simulink model "baitap"  (R2018a)
settings: Solver=ode5  StartTime=0.0  StopTime=3  FixedStep=0.01  RelTol=1e-3
libraries: fuzblock x1
settings Model: Creator=DELL  LastModifiedBy=DELL

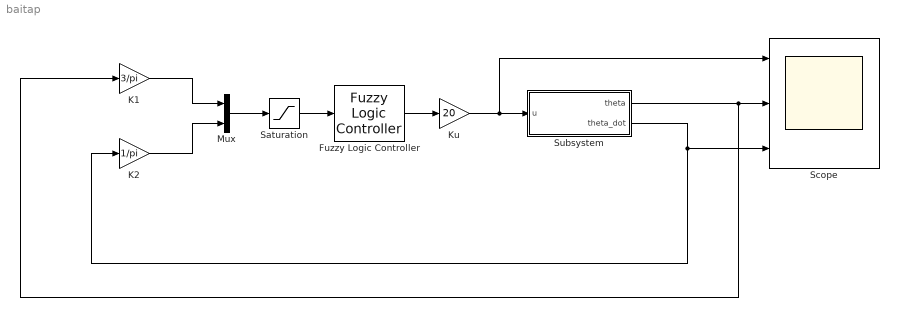
== system baitap ==
  Fuzzy Logic Controller : fuzblock/Fuzzy Logic  Controller  FIS='exex.fis'  OutputSampleNumber=101  DataType=double  FuzzifiedInputs=off  RuleFiringStrengths=off  RuleOutputs=off  AggregatedOutputs=off  SimulateUsing=Interpreted execution  OutOfRangeInputValueMessage=warning  NoRuleFiredMessage=warning  EmptyOutputFuzzySetMessage=warning
  "K1 " : Gain  Gain=3/pi
  "K2 " : Gain  Gain=1/pi
  "Ku " : Gain  Gain=20
  Mux : Mux  Inputs=2
  Saturation : Saturate  UpperLimit=1  LowerLimit=-1
  Scope : Scope  NumInputPorts=3
  Subsystem : Subsystem  mask{M1=1, m=0.1, g=9.81, l=0.5, theta_0=5, theta_dot_0=0}
      mask prompts: theta_0 "theta"; theta_dot_0 "theta_dot"
  wires:
  Saturation/1 -> Fuzzy Logic Controller/1
  Subsystem/1(theta) -> "K1 "/1, Scope/2
  Subsystem/2(theta_dot) -> Scope/3, "K2 "/1
  Fuzzy Logic Controller/1 -> "Ku "/1
  "Ku "/1 -> Subsystem/1(u), Scope/1
  Mux/1 -> Saturation/1
  "K2 "/1 -> Mux/2
  "K1 "/1 -> Mux/1

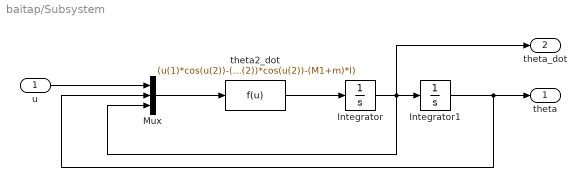
== system baitap/Subsystem ==
  u : Inport
  Integrator : Integrator  InitialCondition=theta_dot_0*pi/180
  Integrator1 : Integrator  InitialCondition=theta_0*pi/180
  Mux : Mux  Inputs=3
  theta2_dot : Fcn  Expr=(u(1)*cos(u(2))-(M1+m)*g*sin(u(2))+m*l*(cos(u(2))*sin(u(2)))*u(3)*u(3))/(m*l*cos(u(2))*cos(u(2))-(M1+m)*l)
  theta : Outport
  theta_dot : Outport  Port=2
  wires:
  theta2_dot/1 -> Integrator/1
  Integrator/1 -> Integrator1/1, Mux/3, theta_dot/1
  Integrator1/1 -> Mux/2, theta/1
  u/1 -> Mux/1
  Mux/1 -> theta2_dot/1
